simulink model "demux_complex_test"  (Simulink 8.4)
settings: Solver=ode45  StartTime=0.0  StopTime=10.0  RelTol=1e-3
settings Model: Creator=arnaud  LastModifiedBy=arnaud
settings DataIOCC: SaveFormat=Structure
settings DebuggingCC: StrictBusMsg=Warning

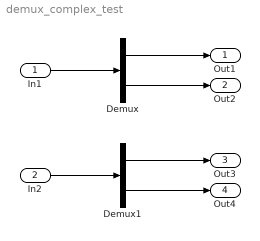
== system demux_complex_test ==
  In1 : Inport
      settings: SignalType=complex
  In2 : Inport  Port=2  PortDimensions=3
      settings: SignalType=complex
  Demux : Demux  Outputs=2
  Demux1 : Demux  Outputs=[1 2]
  Out1 : Outport
  Out2 : Outport  Port=2
  Out3 : Outport  Port=3
  Out4 : Outport  Port=4
  wires:
  In1/1 -> Demux/1
  Demux/1 -> Out1/1
  Demux/2 -> Out2/1
  In2/1 -> Demux1/1
  Demux1/1 -> Out3/1
  Demux1/2 -> Out4/1
